simulink model "atmospheric"  (Simulink 6.1)
settings: Solver=ode45  StartTime=0.0  StopTime=10  RelTol=1e-3
undefined symbols (not defined in the file): Atmospheric, atmospheric_lib
libraries: Accessories_lib x2, exposed_area_lib x1
settings Model: Creator=jala01  LastModifiedBy=Dan T  ExtModeAutoUpdateStatusClock=off
settings DataIOCC: SignalLoggingName=sigsOut
settings HardwareCC: TargetUnknown=on

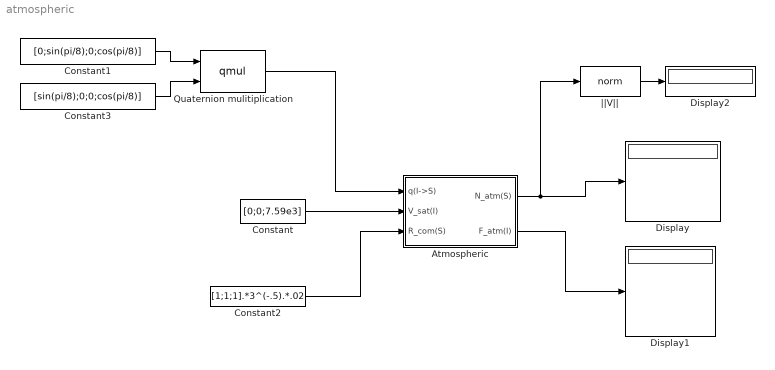
== system atmospheric ==
  Atmospheric : Subsystem  AncestorBlock=atmospheric_lib/Atmospheric
  Constant : Constant  Value=[0;0;7.59e3]
  Constant1 : Constant  Value=[0;sin(pi/8);0;cos(pi/8)]
  Constant2 : Constant  Value=[1;1;1].*3^(-.5).*.02
  Constant3 : Constant  Value=[sin(pi/8);0;0;cos(pi/8)]
  Display : Display
  Display1 : Display
  Display2 : Display
  Quaternion mulitiplication : S-Function  FunctionName=qmul
  ||V|| : MATLABFcn  MATLABFcn=norm
  wires:
  Atmospheric/2(F_atm(I)) -> Display1/1
  Constant1/1 -> Quaternion mulitiplication/1
  Constant3/1 -> Quaternion mulitiplication/2
  ||V||/1 -> Display2/1
  Quaternion mulitiplication/1 -> Atmospheric/1(q(I->S))
  Constant/1 -> Atmospheric/2(V_sat(I))
  Constant2/1 -> Atmospheric/3(R_com(S))
  Atmospheric/1(N_atm(S)) -> Display/1, ||V||/1

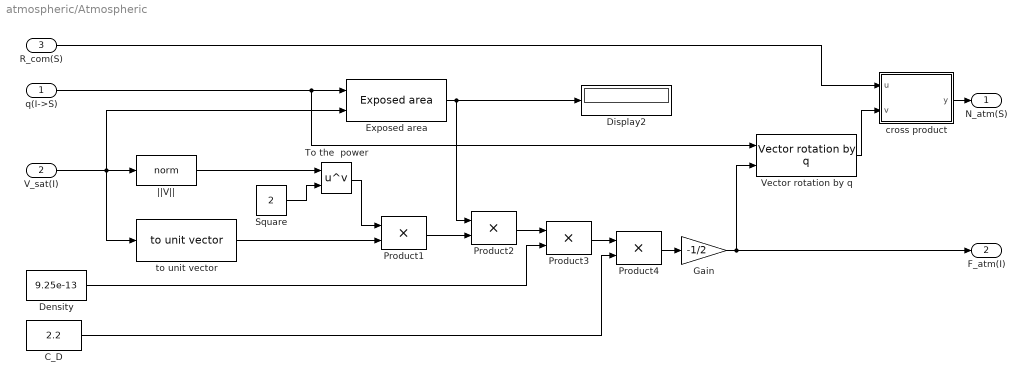
== system atmospheric/Atmospheric ==
  q(I->S) : Inport  Port=1  LatchInput=off
  V_sat(I) : Inport  Port=2  LatchInput=off
  R_com(S) : Inport  Port=3  LatchInput=off
  C_D : Constant  Value=2.2
  Density : Constant  Value=9.25e-13
  Display2 : Display
  Exposed area : exposed_area_lib/Exposed area
  Gain : Gain  Gain=-1/2  SaturateOnIntegerOverflow=on
  Product{1..4} (4 alike) : Product  SaturateOnIntegerOverflow=on
  Square : Constant  Value=2
  To the  power : Math  Operator=pow  SaturateOnIntegerOverflow=on
  Vector rotation by q : Accessories_lib/Math utilities/Vector operations/Vector rotation by q
  cross product : Stateflow chart
  to unit vector : Accessories_lib/Math utilities/Vector operations/to unit vector
  ||V|| : MATLABFcn  MATLABFcn=norm
  N_atm(S) : Outport
  F_atm(I) : Outport  Port=2
  wires:
  cross product/1(y) -> N_atm(S)/1
  Gain/1 -> Vector rotation by q/2, F_atm(I)/1
  Product4/1 -> Gain/1
  q(I->S)/1 -> Vector rotation by q/1, Exposed area/1
  C_D/1 -> Product4/2
  Product3/1 -> Product4/1
  Density/1 -> Product3/2
  Product2/1 -> Product3/1
  Product1/1 -> Product2/2
  To the  power/1 -> Product1/1
  to unit vector/1 -> Product1/2
  ||V||/1 -> To the  power/1
  V_sat(I)/1 -> Exposed area/2, ||V||/1, to unit vector/1
  Exposed area/1 -> Product2/1, Display2/1
  Square/1 -> To the  power/2
  R_com(S)/1 -> cross product/1(u)
  Vector rotation by q/1 -> cross product/2(v)

== matlab function Atmospheric/cross product ==
  data: u input inherited; y output inherited; v input inherited
function y = crossproduct(u,v)
% This block supports an embeddable subset of the MATLAB language.
% See the help menu for details. 

y = [u(2)*v(3)-u(3)*v(2);u(3)*v(1)-u(1)*v(3);u(1)*v(2)-u(2)*v(1)];
